simulink model "ProjetGies"  (R2023b)
settings: Solver=ode15s  StartTime=0.0  StopTime=11  MaxStep=0.22  RelTol=1e-3
InitFcn:
  | ProjetGiesData
values from neighbouring files (symbols this model uses):
  f = 0.8    [ProjetGiesData.m]
  J = 3.2284E-6    (= 3.2284e-06)    [MCC_constants.m]    (also in ProjetGiesData.m = 0.5; Td2.m = 0.28; Tp3_data.m = 0.2)
  m = 1000    [ProjetGiesData.m]
  N = m*g/4    (= 2452.5)    [ProjetGiesData.m]
  rRoue = 0.3    [ProjetGiesData.m]
  v0 = 100    [ProjetGiesData.m]
libraries: simulink x2
settings Model: Creator=Table2  LastModifiedBy=yannm
settings SolverCC: AlgebraicLoopSolver=TrustRegion
settings DataIOCC: ReturnWorkspaceOutputs=off
settings DebuggingCC: UnconnectedInputMsg=warning  UnconnectedOutputMsg=warning  UnconnectedLineMsg=warning  ArithmeticOperatorsInVariantConditions=warning
settings ModelReferenceCC: EnableRefExpFcnMdlSchedulingChecks=on
settings SFSimCC: SimUseLocalCustomCode=off  CustomCodeUndefinedFunction=UseInterfaceOnly
settings RTWCC: RTWUseLocalCustomCode=off

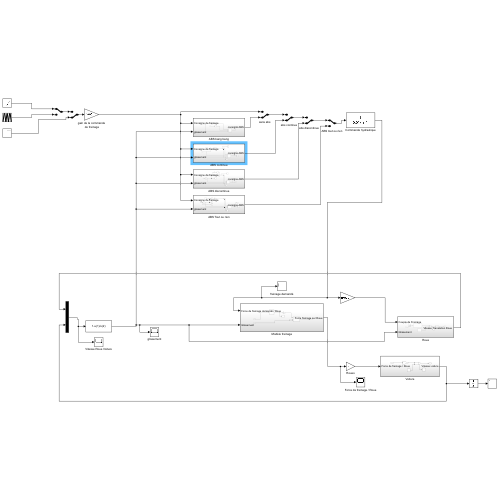
[thumbnail: Simulink's stored preview of the top-level diagram]
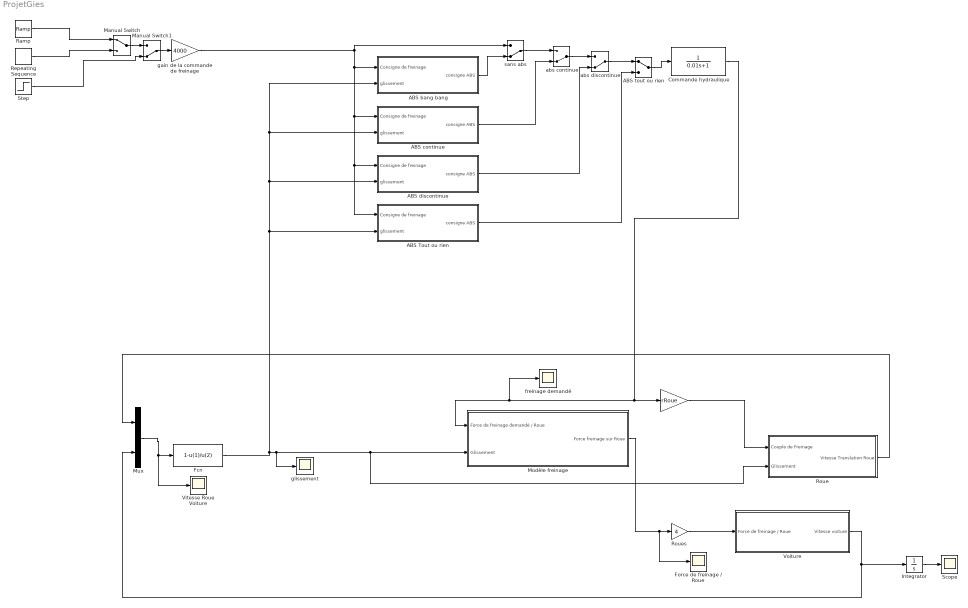
== system ProjetGies ==
  " " : Gain  Gain=rRoue
  ABS Tout ou rien : Subsystem
  ABS bang bang : Subsystem
  ABS continue : Subsystem
  ABS discontinue : Subsystem
  ABS tout ou rien : ManualSwitch
  Commande hydraulique : TransferFcn  Denominator=[0.01 1]
  Fcn : Fcn  Expr=1-u(1)/u(2)
  "Force de freinage / Roue " : Scope
  Integrator : Integrator
  Manual Switch : ManualSwitch
  Manual Switch1 : ManualSwitch  CurrentSetting=0
  "Modèle freinage " : Subsystem
  Mux : Mux  Inputs=2
  Ramp : simulink/Sources/Ramp  slope=2  start=0  InitialOutput=0
  Repeating Sequence : simulink/Sources/Repeating Sequence  rep_seq_t=[0 2 3 5]  rep_seq_y=[0 1 1 0]
  "Roue " : Subsystem
  "Roues " : Gain  Gain=4
  Scope : Scope
  Step : Step  Time=0.5  SampleTime=0
  "Vitesse Roue Voiture " : Scope
  "Voiture " : Subsystem
  abs continue : ManualSwitch  CurrentSetting=0
  abs discontinue : ManualSwitch  CurrentSetting=0
  freinage demandé : Scope
  "gain de la commande de freinage " : Gain  Gain=4000
  glissement : Scope
  sans abs : ManualSwitch  CurrentSetting=0
  wires:
  "Roues "/1 -> "Voiture "/1("Force de freinage / Roue ")
  "Modèle freinage "/1(Force freinage sur Roue) -> "Force de freinage / Roue "/1, "Roues "/1
  " "/1 -> "Roue "/1("Couple de Freinage ")
  "Roue "/1("Vitesse Translation Roue ") -> Mux/1
  "Voiture "/1(Vitesse voiture) -> Mux/2, Integrator/1
  Mux/1 -> "Vitesse Roue Voiture "/1, Fcn/1
  Repeating Sequence/1 -> Manual Switch/2
  Ramp/1 -> Manual Switch/1
  Step/1 -> Manual Switch1/2
  Manual Switch/1 -> Manual Switch1/1
  Manual Switch1/1 -> "gain de la commande de freinage "/1
  Integrator/1 -> Scope/1
  Fcn/1 -> ABS Tout ou rien/2(glissement), ABS continue/2(glissement), ABS bang bang/2(glissement), ABS discontinue/2(glissement), glissement/1, "Modèle freinage "/2(Glissement), "Roue "/2("Glissement ")
  "gain de la commande de freinage "/1 -> ABS Tout ou rien/1(Consigne de freinage), ABS discontinue/1(Consigne de freinage), ABS continue/1(Consigne de freinage), ABS bang bang/1(Consigne de freinage), sans abs/1
  Commande hydraulique/1 -> " "/1, "Modèle freinage "/1("Force de freinage demandé / Roue "), freinage demandé/1
  ABS bang bang/1(consigne ABS) -> sans abs/2
  ABS continue/1(consigne ABS) -> abs continue/2
  sans abs/1 -> abs continue/1
  ABS discontinue/1(consigne ABS) -> abs discontinue/2
  abs continue/1 -> abs discontinue/1
  abs discontinue/1 -> ABS tout ou rien/1
  ABS tout ou rien/1 -> Commande hydraulique/1
  ABS Tout ou rien/1(consigne ABS) -> ABS tout ou rien/2

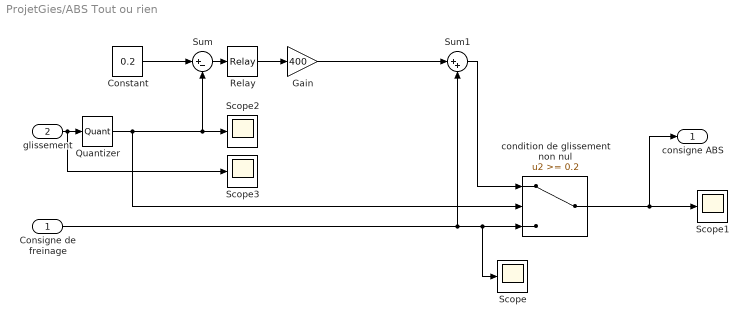
== system ProjetGies/ABS Tout ou rien ==
  Consigne de freinage : Inport
  glissement : Inport  Port=2
  Constant : Constant  Value=0.2
  Gain : Gain  Gain=400
  Quantizer : Quantizer  QuantizationInterval=1/10000  LinearizeAsGain=off
  Relay : Relay  OnSwitchValue=0  OffSwitchValue=0  OffOutputValue=-1
  Scope{,1..3} (4 alike) : Scope
  Sum : Sum  Inputs=|+-
  Sum1 : Sum  Inputs=|++
  condition de glissement non nul : Switch  Threshold=0.2  SaturateOnIntegerOverflow=off  InputSameDT=off
  consigne ABS : Outport
  wires:
  Consigne de freinage/1 -> Sum1/2, Scope/1, condition de glissement non nul/3
  condition de glissement non nul/1 -> Scope1/1, consigne ABS/1
  Constant/1 -> Sum/1
  glissement/1 -> Scope3/1, Quantizer/1
  Sum1/1 -> condition de glissement non nul/1
  Quantizer/1 -> condition de glissement non nul/2, Sum/2, Scope2/1
  Sum/1 -> Relay/1
  Relay/1 -> Gain/1
  Gain/1 -> Sum1/1

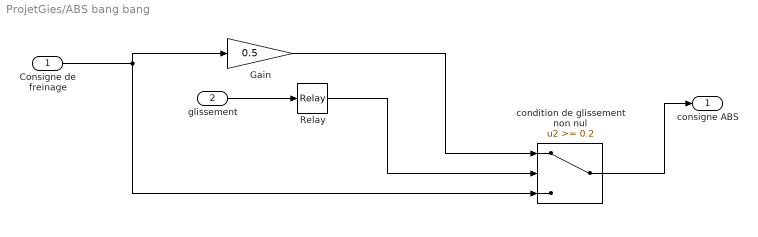
== system ProjetGies/ABS bang bang ==
  Consigne de freinage : Inport
  glissement : Inport  Port=2
  Gain : Gain  Gain=0.5
  Relay : Relay  OnSwitchValue=0.2001  OffSwitchValue=0.1999
  condition de glissement non nul : Switch  Threshold=0.2  SaturateOnIntegerOverflow=off  InputSameDT=off
  consigne ABS : Outport
  wires:
  Consigne de freinage/1 -> condition de glissement non nul/3, Gain/1
  glissement/1 -> Relay/1
  Relay/1 -> condition de glissement non nul/2
  condition de glissement non nul/1 -> consigne ABS/1
  Gain/1 -> condition de glissement non nul/1

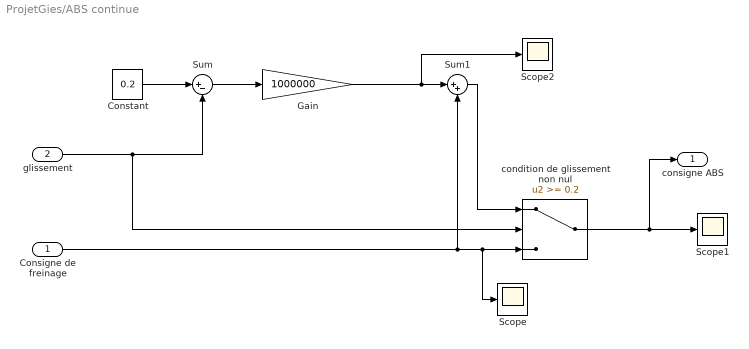
== system ProjetGies/ABS continue ==
  Consigne de freinage : Inport
  glissement : Inport  Port=2
  Constant : Constant  Value=0.2
  Gain : Gain  Gain=1000000
  Scope : Scope
  Scope1 : Scope
  Scope2 : Scope
  Sum : Sum  Inputs=|+-
  Sum1 : Sum  Inputs=|++
  condition de glissement non nul : Switch  Threshold=0.2  SaturateOnIntegerOverflow=off  InputSameDT=off
  consigne ABS : Outport
  wires:
  Consigne de freinage/1 -> Sum1/2, Scope/1, condition de glissement non nul/3
  condition de glissement non nul/1 -> Scope1/1, consigne ABS/1
  Constant/1 -> Sum/1
  Sum/1 -> Gain/1
  Sum1/1 -> condition de glissement non nul/1
  glissement/1 -> condition de glissement non nul/2, Sum/2
  Gain/1 -> Scope2/1, Sum1/1

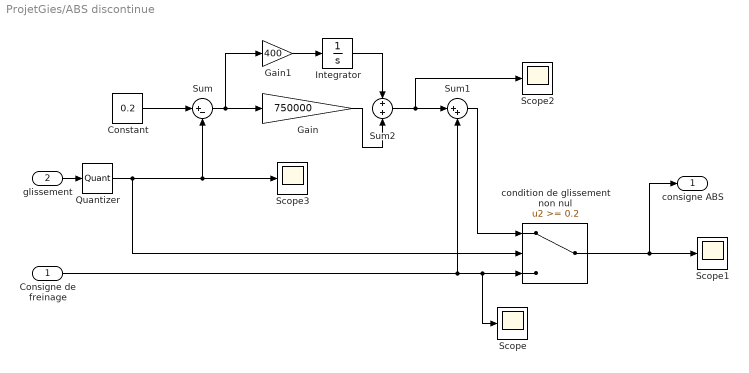
== system ProjetGies/ABS discontinue ==
  Consigne de freinage : Inport
  glissement : Inport  Port=2
  Constant : Constant  Value=0.2
  Gain : Gain  Gain=750000
  Gain1 : Gain  Gain=400
  Integrator : Integrator
  Quantizer : Quantizer  QuantizationInterval=1/10000
  Scope{,1..3} (4 alike) : Scope
  Sum : Sum  Inputs=|+-
  Sum1 : Sum  Inputs=|++
  Sum2 : Sum  Inputs=+|+
  condition de glissement non nul : Switch  Threshold=0.2  SaturateOnIntegerOverflow=off  InputSameDT=off
  consigne ABS : Outport
  wires:
  Consigne de freinage/1 -> Sum1/2, Scope/1, condition de glissement non nul/3
  condition de glissement non nul/1 -> Scope1/1, consigne ABS/1
  Constant/1 -> Sum/1
  glissement/1 -> Quantizer/1
  Sum/1 -> Gain1/1, Gain/1
  Sum1/1 -> condition de glissement non nul/1
  Quantizer/1 -> condition de glissement non nul/2, Sum/2, Scope3/1
  Gain/1 -> Sum2/2
  Sum2/1 -> Scope2/1, Sum1/1
  Integrator/1 -> Sum2/1
  Gain1/1 -> Integrator/1

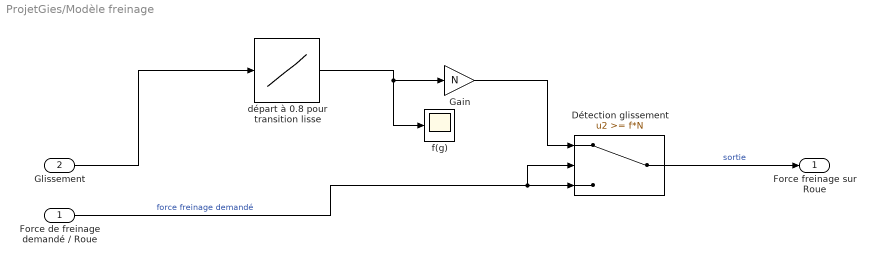
== system ProjetGies/Modèle freinage  ==
  "Force de freinage demandé / Roue " : Inport
  Glissement : Inport  Port=2
  "Détection glissement " : Switch  Threshold=f*N  SaturateOnIntegerOverflow=off  InputSameDT=off
  Gain : Gain  Gain=N
  départ à 0.8 pour transition lisse : Lookup_n-D  NumberOfTableDimensions=1  BreakpointsForDimension1=[0,0.1,0.15,0.2,0.3,0.4,0.5,0.6,0.7,0.8,0.9,1]  Table=[0.8,0.85,0.9,0.95,0.8,0.73,0.69,0.66,0.65,0.64,0.62,0.61]  InternalRulePriority=Speed  RndMeth=Simplest
  "f(g) " : Scope
  Force freinage sur Roue : Outport  VectorParamsAs1DForOutWhenUnconnected=off
  wires:
  "Détection glissement "/1 -> Force freinage sur Roue/1  "sortie"
  Glissement/1 -> départ à 0.8 pour transition lisse/1
  "Force de freinage demandé / Roue "/1 -> "Détection glissement "/2, "Détection glissement "/3  "force freinage demandé"
  départ à 0.8 pour transition lisse/1 -> "f(g) "/1, Gain/1
  Gain/1 -> "Détection glissement "/1

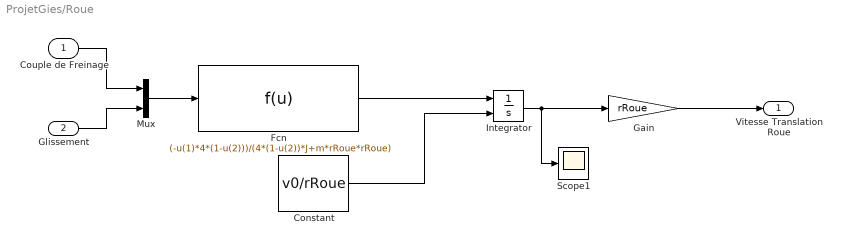
== system ProjetGies/Roue  ==
  "Couple de Freinage " : Inport
  "Glissement " : Inport  Port=2
  Constant : Constant  Value=v0/rRoue
  Fcn : Fcn  Expr=(-u(1)*4*(1-u(2)))/(4*(1-u(2))*J+m*rRoue*rRoue)
  Gain : Gain  Gain=rRoue
  Integrator : Integrator  InitialConditionSource=external  LimitOutput=on  LowerSaturationLimit=0
  Mux : Mux  Inputs=2
  Scope1 : Scope
  "Vitesse Translation Roue " : Outport  VectorParamsAs1DForOutWhenUnconnected=off
  wires:
  Mux/1 -> Fcn/1
  "Glissement "/1 -> Mux/2
  Fcn/1 -> Integrator/1
  Constant/1 -> Integrator/2
  Integrator/1 -> Gain/1, Scope1/1
  Gain/1 -> "Vitesse Translation Roue "/1
  "Couple de Freinage "/1 -> Mux/1

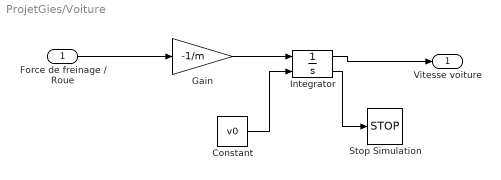
== system ProjetGies/Voiture  ==
  "Force de freinage / Roue " : Inport
  Constant : Constant  Value=v0
  Gain : Gain  Gain=-1/m
  Integrator : Integrator  InitialConditionSource=external  LimitOutput=on  UpperSaturationLimit=150  LowerSaturationLimit=0.0001  ShowSaturationPort=on
  Stop Simulation : Stop
  Vitesse voiture : Outport  VectorParamsAs1DForOutWhenUnconnected=off
  wires:
  "Force de freinage / Roue "/1 -> Gain/1
  Constant/1 -> Integrator/2
  Gain/1 -> Integrator/1
  Integrator/1 -> Vitesse voiture/1
  Integrator/2 -> Stop Simulation/1
